simulink model "SIM_sliding_double_pendulum"  (R2020b)
settings: Solver=ode4  StartTime=0.0  StopTime=5  RelTol=1e-3
values from neighbouring files (symbols this model uses):
  g = 9.81    [SIM_sliding_double_pendulum_init.m]
  l1 = 0.379    [SIM_sliding_double_pendulum_init.m]
  l2 = 0.315    [SIM_sliding_double_pendulum_init.m]
  m1 = 0.5    [SIM_sliding_double_pendulum_init.m]
  m2 = 0.536    [SIM_sliding_double_pendulum_init.m]
  m3 = 0.176    [SIM_sliding_double_pendulum_init.m]
  teta1_init = 0*pi/180    (= 0)    [SIM_sliding_double_pendulum_init.m]
  teta2_init = 0.5*pi/180    (= 0.00872664625997)    [SIM_sliding_double_pendulum_init.m]
  x_init = 0    [SIM_sliding_double_pendulum_init.m]
libraries: pid_lib x1
settings Model: Creator=Yigit  LastModifiedBy=Yigit

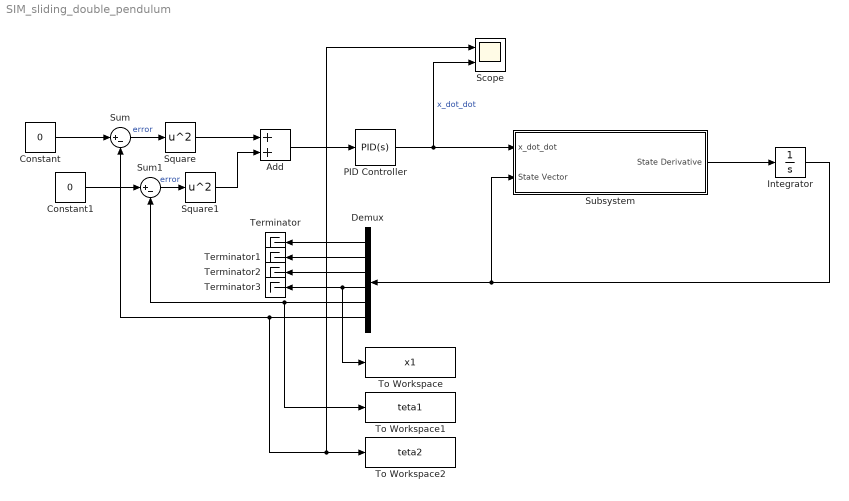
== system SIM_sliding_double_pendulum ==
  Add : Sum
  Constant : Constant  Value=0
  Constant1 : Constant  Value=0
  Demux : Demux  Outputs=6
  Integrator : Integrator  InitialCondition=[0;0;0;x_init;teta1_init;teta2_init]
  PID Controller : pid_lib/PID Controller  Controller=PID  Form=Parallel  TimeDomain=Continuous-time  UseExternalTs=off  SampleTime=-1  IntegratorMethod=Forward Euler  FilterMethod=Forward Euler  ControllerParametersSource=internal  P=1  I=1  D=1  UseFilter=on  N=1  TunerSelectOption=Transfer Function Based (PID Tuner App)  InitialConditionSource=internal  InitialConditionForIntegrator=0  InitialConditionForFilter=0  DifferentiatorICPrevScaledInput=0  ExternalReset=none  TrackingMode=off  Kt=1  LimitOutput=off  SatLimitsSource=internal  UpperSaturationLimit=inf  LowerSaturationLimit=-inf  LinearizeAsGain=on  AntiWindupMode=none  Kb=1  POutMin=[]  POutMax=[]  IOutMin=[]  IOutMax=[]  DOutMin=[]  DOutMax=[]  NOutMin=[]  NOutMax=[]  SumOutMin=[]  SumOutMax=[]  SaturationOutMin=[]  SaturationOutMax=[]  PParamMin=[]  PParamMax=[]  IParamMin=[]  IParamMax=[]  DParamMin=[]  DParamMax=[]  NParamMin=[]  NParamMax=[]  KbParamMin=[]  KbParamMax=[]  KtParamMin=[]  KtParamMax=[]  KbOutMin=[]  KbOutMax=[]  KtOutMin=[]  KtOutMax=[]  IntegratorOutMin=[]  IntegratorOutMax=[]  FilterOutMin=[]  FilterOutMax=[]  SumI1OutMin=[]  SumI1OutMax=[]  SumI2OutMin=[]  SumI2OutMax=[]  SumI3OutMin=[]  SumI3OutMax=[]  SumI4OutMin=[]  SumI4OutMax=[]  SumDOutMin=[]  SumDOutMax=[]  DifferentiatorOutMin=[]  DifferentiatorOutMax=[]  FilterDiffOutCoefMin=[]  FilterDiffOutCoefMax=[]  ReciprocalOutMin=[]  ReciprocalOutMax=[]  SumDenOutMin=[]  SumDenOutMax=[]  SumNumOutMin=[]  SumNumOutMax=[]  DivideOutMin=[]  DivideOutMax=[]  UdiffTsProdOutMin=[]  UdiffTsProdOutMax=[]  NTsProdOutMin=[]  NTsProdOutMax=[]  UintegralTsProdOutMin=[]  UintegralTsProdOutMax=[]  UngainTsProdOutMin=[]  UngainTsProdOutMax=[]  IntegratorContinuousStateAttributes=''  IntegratorStateMustResolveToSignalObject=off  IntegratorRTWStateStorageClass=Auto  FilterContinuousStateAttributes=''  FilterStateMustResolveToSignalObject=off  FilterRTWStateStorageClass=Auto  ParallelPVariant=InternalParameters  IdealPVariant=Disabled  IVariant=InternalParameters  DVariant=InternalParameters  IntegratorVariant=Continuous  SatVariant=Disabled  AWVariant=Passthrough  PCopyVariant=Disabled  TRVariant=Disabled  FdbkBlocksVariant=Forward  IdealPFdbkVariant=Disabled  SatFdbkVariant=Disabled  DerivativeFilterVariant=ContFilter  NVariant=InternalParameters  NCopyVariant=Disabled  FilterICVariant=InternalICsFilter  IntegratorICVariant=InternalICs  ExternalResetVariant=Disabled  TRSumVariant=Passthrough  SumFdbkVariant=Disabled  SumVariant=Sum_PID  TsampFilterVariant=InternalTs  TsampNgainVariant=Passthrough  TsampIntegralVariant=Passthrough  ExternalSaturationOutDataTypeStr=Inherit: Same as second input
  Scope : Scope  NumInputPorts=2
  Square : Math  Operator=square  SaturateOnIntegerOverflow=on
  Square1 : Math  Operator=square  SaturateOnIntegerOverflow=on
  Subsystem : Subsystem
  Sum : Sum  Inputs=|+-
  Sum1 : Sum  Inputs=|+-
  Terminator{,1..3} (4 alike) : Terminator
  To Workspace : ToWorkspace  VariableName=x1  SaveFormat=Timeseries  SampleTime=-1
  To Workspace1 : ToWorkspace  VariableName=teta1  SaveFormat=Timeseries  SampleTime=-1
  To Workspace2 : ToWorkspace  VariableName=teta2  SaveFormat=Timeseries  SampleTime=-1
  wires:
  Subsystem/1(State Derivative) -> Integrator/1
  Integrator/1 -> Subsystem/2(State Vector), Demux/1
  Constant/1 -> Sum/1
  Demux/6 -> Scope/1, To Workspace2/1, Sum/2
  Demux/1 -> Terminator/1
  Demux/2 -> Terminator1/1
  Demux/3 -> Terminator2/1
  Demux/4 -> To Workspace/1, Terminator3/1
  Demux/5 -> Sum1/2, To Workspace1/1
  Constant1/1 -> Sum1/1
  Sum/1 -> Square/1  "error"
  Sum1/1 -> Square1/1  "error"
  Square/1 -> Add/1
  Square1/1 -> Add/2
  Add/1 -> PID Controller/1
  PID Controller/1 -> Scope/2, Subsystem/1(x_dot_dot)  "x_dot_dot"

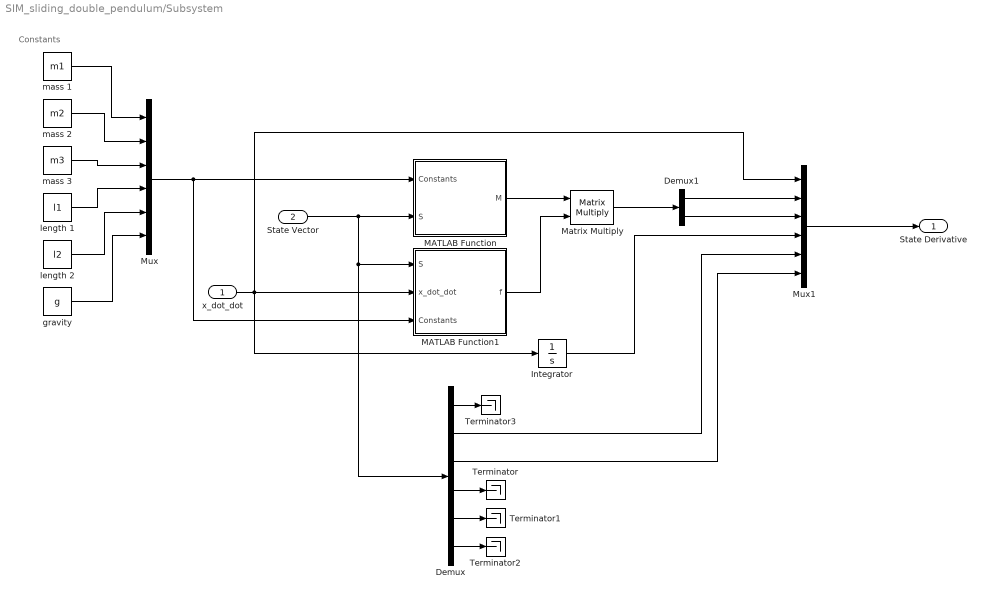
== system SIM_sliding_double_pendulum/Subsystem ==
  note: Constants
  x_dot_dot : Inport
  State Vector : Inport  Port=2
  Demux : Demux  Outputs=6
  Demux1 : Demux  Outputs=2
  Integrator : Integrator
  MATLAB Function : MATLAB Function  TreatAsAtomicUnit=on
  MATLAB Function1 : MATLAB Function  TreatAsAtomicUnit=on
  Matrix Multiply : Product  Multiplication=Matrix(*)
  Mux : Mux  Inputs=6
  Mux1 : Mux  Inputs=6
  Terminator{,1..3} (4 alike) : Terminator
  gravity : Constant  Value=g
  length 1 : Constant  Value=l1
  length 2 : Constant  Value=l2
  mass 1 : Constant  Value=m1
  mass 2 : Constant  Value=m2
  mass 3 : Constant  Value=m3
  State Derivative : Outport
  wires:
  State Vector/1 -> Demux/1, MATLAB Function1/1(S), MATLAB Function/2(S)
  MATLAB Function1/1(f) -> Matrix Multiply/2
  MATLAB Function/1(M) -> Matrix Multiply/1
  mass 1/1 -> Mux/1
  mass 2/1 -> Mux/2
  mass 3/1 -> Mux/3
  length 1/1 -> Mux/4
  length 2/1 -> Mux/5
  gravity/1 -> Mux/6
  Mux/1 -> MATLAB Function1/3(Constants), MATLAB Function/1(Constants)
  Mux1/1 -> State Derivative/1
  Demux/4 -> Terminator/1
  Demux/5 -> Terminator1/1
  Demux/6 -> Terminator2/1
  x_dot_dot/1 -> Integrator/1, Mux1/1, MATLAB Function1/2(x_dot_dot)
  Matrix Multiply/1 -> Demux1/1
  Demux1/1 -> Mux1/2
  Demux1/2 -> Mux1/3
  Demux/2 -> Mux1/5
  Demux/3 -> Mux1/6
  Integrator/1 -> Mux1/4
  Demux/1 -> Terminator3/1

== matlab function SIM_sliding_double_pendulum/Subsystem/MATLAB Function ==
  data: Constants input; S input; M output
function M = Minv( Constants,S) %inverse mass matrix
m1 = Constants(1) ;
m2 = Constants(2) ;
m3 = Constants(3) ;
l1 = Constants(4) ;
l2 = Constants(5) ;
% M = inv([ (m1+m2+m3)  (m2*l1*cos(S(5))+m3*l1*cos(S(5)))  (m3*l2*cos(S(6)));
%           ((m2+m3)*l1*cos(S(5)))  ((m2+m3)*(l1^2))  (m3*l1*l2*cos(S(5)-S(6))); 
%           (m3*l2*cos(S(6)))  (m3*l1*l2*cos(S(5)-S(6)))  (m3*(l2^2))       ]) ;


M = inv([ ((m2+m3)*(l1^2))  (m3*l1*l2*cos(S(5)-S(6))); 
          (m3*l1*l2*cos(S(5)-S(6)))  (m3*(l2^2))       ]) ;

== matlab function SIM_sliding_double_pendulum/Subsystem/MATLAB Function1 ==
  data: S input; f output; x_dot_dot input; Constants input
function f = F(S, x_dot_dot, Constants)
m1 = Constants(1) ;
m2 = Constants(2) ;
m3 = Constants(3) ;
l1 = Constants(4) ;
l2 = Constants(5) ;
g  = Constants(6) ;
% f = [ (m2+m3)*l1*(S(2)^2)*sin(S(5)) + m3*l2*(S(6)^2)*sin(S(6))+Force;
%       (m2+m3)*l1*g*sin(S(5)) - m3*l1*l2*(S(6)^2)*sin(S(5)-S(6));
%       (m3*g*l2*sin(S(6)) + m3*l1*l2*(S(5)^2)*sin(S(5)-S(6)) ) ] ;

f = [ (m2+m3)*l1*g*sin(S(5)) - m3*l1*l2*(S(6)^2)*sin(S(5)-S(6)) - x_dot_dot*((m2+m3)*l1*cos(S(5)))  ;
      (m3*g*l2*sin(S(6)) + m3*l1*l2*(S(5)^2)*sin(S(5)-S(6)) - x_dot_dot*(m3*l2*cos(S(6)))   ) ] ;
